simulink model "mpsk_model_inclass"  (R2022a)
settings: Solver=VariableStepAuto  StartTime=0.0  StopTime=10.0  RelTol=1e-3
values from neighbouring files (symbols this model uses):
  Tb = 1/Rb    (= 0.0001)    [mfsk_sim.m]    (also in mpam_mqam_compare.m = 1/Rb_mqam; mpam_sim.m = 1/Rb; mpsk_sim.m = 1/Rb; mqam_mpsk_compare.m = 1/Rb_mqam)
libraries: simulink x2, commdigbbndpm3 x2, commchan3 x1, commrandsrc3 x1, commsink2 x1
settings Model: Creator=ozand  LastModifiedBy=ozand

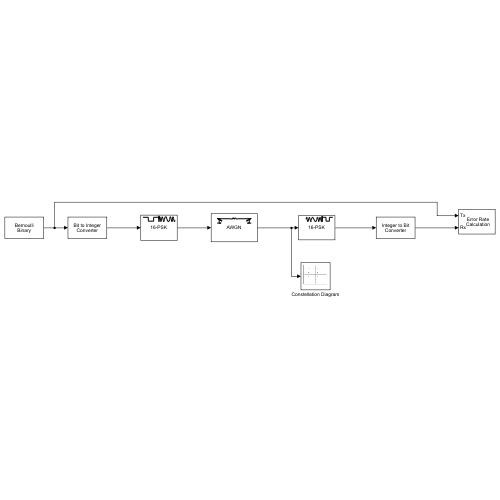
[thumbnail: Simulink's stored preview of the top-level diagram]
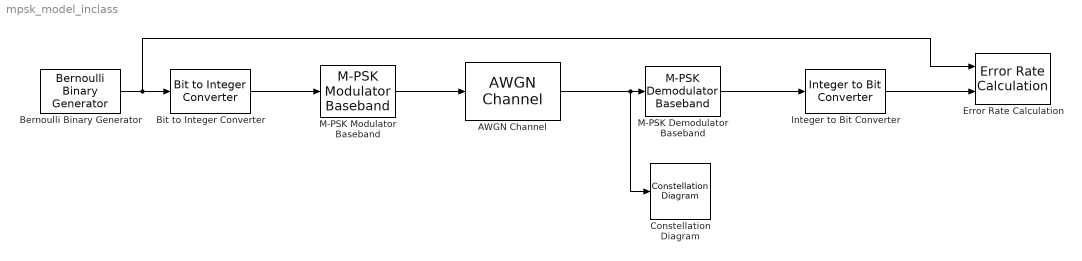
== system mpsk_model_inclass ==
  AWGN Channel : commchan3/AWGN Channel  InputProcessing=Columns as channels (frame based)  seed=67  noiseMode="Signal to noise ratio  (Eb/No)"  EbNodB=EbN0dB  EsNodB=10  SNRdB=10  bitsPerSym=k  Ps=1  Tsym=Ts  variance=1
  Bernoulli Binary Generator : commrandsrc3/Bernoulli Binary Generator  ProbabilityOfZero=0.5  SeedSource=Auto  Seed=0  SampleTime=Tb  SamplesPerFrame=3600  OutputDataType=double  SimulateUsing=Interpreted execution
  Bit to Integer Converter : simulink/Logic and Bit Operations/Bit to Integer Converter  nbits=k  bitOrder=MSB first  signedOutputValues=Unsigned  outDtype=Inherit via internal rule  outDtypeSigned=Inherit via internal rule
      settings: SourceProductBaseCode=SL
  Constellation Diagram : ConstellationDiagram  WindowPosition=[699.000000,81.000000,806.000000,683.000000,]  Visible=on  ScopeFrameLocation=window  DefaultConfigurationName=comm.scopes.ConstellationDiagramBlockCfg
  Error Rate Calculation : commsink2/Error Rate Calculation  N=0  st_delay=0  cp_mode=Entire frame  subframe=[]  PMode=Workspace  WsName=ErrorVec  RsMode2=off  stop=off  numErr=100  maxBits=1e6
  Integer to Bit Converter : simulink/Logic and Bit Operations/Integer to Bit Converter  nbits=k  signedInputValues=Unsigned  bitOrder=MSB first  outDtype=Inherit via internal rule
      settings: SourceProductBaseCode=SL
  M-PSK Demodulator Baseband : commdigbbndpm3/M-PSK Demodulator Baseband  M=M  OutType=Integer  DecType=Hard decision  VarSource=Dialog  Variance=1  Dec=Gray  Mapping=[0:7]  Ph=0  outDtype1=Inherit via internal rule  outDtype2=Inherit via internal rule  derotateFactorWordLen=16  derotateFactorDataTypeStr=Inherit: Same word length as input  derotateFactorLastDataTypeStr=Inherit: Same word length as input
  M-PSK Modulator Baseband : commdigbbndpm3/M-PSK Modulator Baseband  M=M  InType=Integer  Enc=Gray  Mapping=[0:7]  Ph=0  outDtype=double  outWordLen=16  outUDDataType=sfix(16)  outFracLenMode=Best precision  outFracLen=15  outDataTypeStr=double  outLastDataTypeStr=double
  wires:
  Bernoulli Binary Generator/1 -> Error Rate Calculation/1, Bit to Integer Converter/1
  Bit to Integer Converter/1 -> M-PSK Modulator Baseband/1
  M-PSK Modulator Baseband/1 -> AWGN Channel/1
  AWGN Channel/1 -> M-PSK Demodulator Baseband/1, Constellation Diagram/1
  M-PSK Demodulator Baseband/1 -> Integer to Bit Converter/1
  Integer to Bit Converter/1 -> Error Rate Calculation/2
